simulink model "imuentiljorgen"  (R2024a)
settings: Solver=VariableStepAuto  StartTime=0.0  StopTime=inf  RelTol=1e-3
StopFcn:
  | send_score(1.1,200);
libraries: read x2, init x1
settings Model: Creator=adriaeik  LastModifiedBy=adriaeik

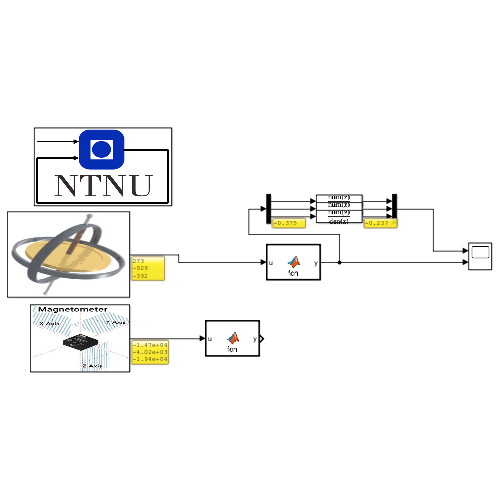
[thumbnail: Simulink's stored preview of the top-level diagram]
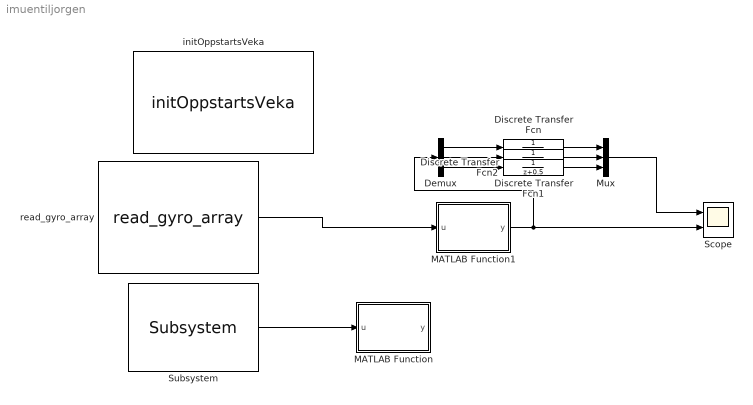
== system imuentiljorgen ==
  Demux : Demux  Outputs=3
  Discrete Transfer Fcn : DiscreteTransferFcn
  Discrete Transfer Fcn1 : DiscreteTransferFcn
  Discrete Transfer Fcn2 : DiscreteTransferFcn
  MATLAB Function : MATLAB Function  TreatAsAtomicUnit=on
  MATLAB Function1 : MATLAB Function  TreatAsAtomicUnit=on
  Mux : Mux  Inputs=3
  Scope : Scope  NumInputPorts=2
  Subsystem : read/Subsystem
  initOppstartsVeka : init/initOppstartsVeka  carID=14  groupID=43
  read_gyro_array : read/read_gyro_array
  wires:
  read_gyro_array/1 -> MATLAB Function1/1(u)
  Subsystem/1 -> MATLAB Function/1(u)
  MATLAB Function1/1(y) -> Demux/1, Scope/2
  Demux/1 -> Discrete Transfer Fcn/1
  Demux/2 -> Discrete Transfer Fcn1/1
  Demux/3 -> Discrete Transfer Fcn2/1
  Discrete Transfer Fcn/1 -> Mux/1
  Discrete Transfer Fcn1/1 -> Mux/2
  Discrete Transfer Fcn2/1 -> Mux/3
  Mux/1 -> Scope/1

== matlab function imuentiljorgen/MATLAB Function ==
  data: u input; y output
function y = fcn(u)
u = u(:);
y = u/norm(u);

== matlab function imuentiljorgen/MATLAB Function1 ==
  data: u input; y output
function y = fcn(u)
u = u(:);
y = u/norm(u);
